simulink model "EM_3"  (R2016a)
settings: Solver=VariableStepAuto  StartTime=0.0  StopTime=0.12  RelTol=1e-3
settings Model: Creator=Максим  LastModifiedBy=Максим

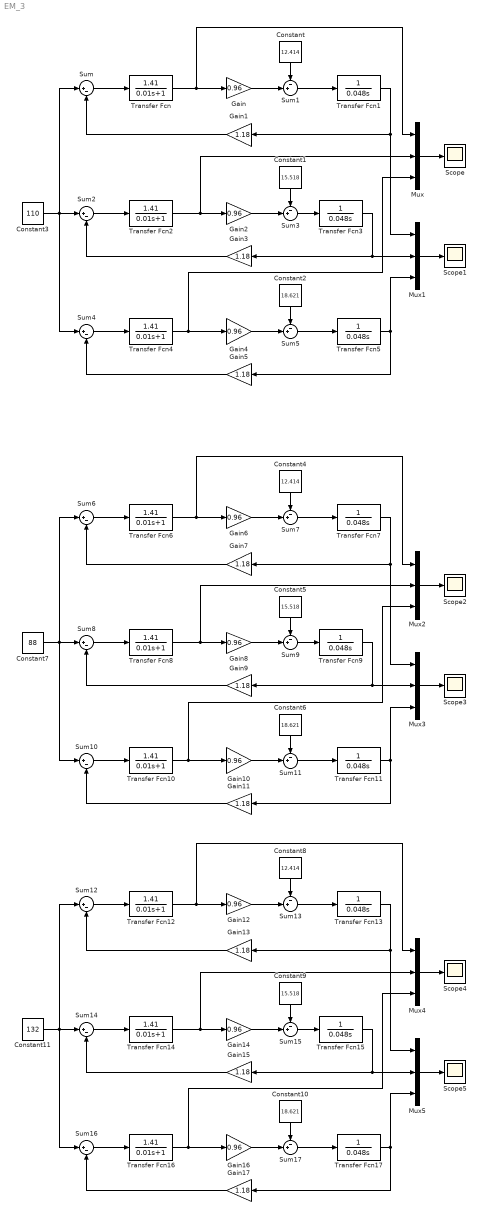
== system EM_3 ==
  Constant : Constant  Value=12.414
  Constant1 : Constant  Value=15.518
  Constant10 : Constant  Value=18.621
  Constant11 : Constant  Value=132
  Constant2 : Constant  Value=18.621
  Constant3 : Constant  Value=110
  Constant4 : Constant  Value=12.414
  Constant5 : Constant  Value=15.518
  Constant6 : Constant  Value=18.621
  Constant7 : Constant  Value=88
  Constant8 : Constant  Value=12.414
  Constant9 : Constant  Value=15.518
  Gain{,2,4,6,8,10,12,14,16} (9 alike) : Gain  Gain=0.96
  Gain{1,3,5,7,9,11,13,15,17} (9 alike) : Gain  Gain=1.18
  Mux{,1..5} (6 alike) : Mux  Inputs=3
  Scope{,1..5} (6 alike) : Scope
  Sum{,2,4,6,8,10,12,14,16} (9 alike) : Sum  Inputs=|+-
  Sum{1,3,5,7,9,11,13,15,17} (9 alike) : Sum  Inputs=-+|
  Transfer Fcn{,2,4,6,8,10,12,14,16} (9 alike) : TransferFcn  Numerator=[1.41]  Denominator=[0.01 1]
  Transfer Fcn{1,3,5,7,9,11,13,15,17} (9 alike) : TransferFcn  Denominator=[0.048 0]
  wires:
  Sum1/1 -> Transfer Fcn1/1
  Constant/1 -> Sum1/1
  Gain/1 -> Sum1/2
  Transfer Fcn/1 -> Mux/1, Gain/1
  Sum/1 -> Transfer Fcn/1
  Transfer Fcn1/1 -> Mux1/1, Gain1/1
  Gain1/1 -> Sum/2
  Sum3/1 -> Transfer Fcn3/1
  Constant1/1 -> Sum3/1
  Gain2/1 -> Sum3/2
  Transfer Fcn2/1 -> Mux/2, Gain2/1
  Sum2/1 -> Transfer Fcn2/1
  Transfer Fcn3/1 -> Mux1/2, Gain3/1
  Gain3/1 -> Sum2/2
  Sum5/1 -> Transfer Fcn5/1
  Constant2/1 -> Sum5/1
  Gain4/1 -> Sum5/2
  Transfer Fcn4/1 -> Mux/3, Gain4/1
  Sum4/1 -> Transfer Fcn4/1
  Transfer Fcn5/1 -> Gain5/1, Mux1/3
  Gain5/1 -> Sum4/2
  Constant3/1 -> Sum2/1, Sum/1, Sum4/1
  Mux/1 -> Scope/1
  Mux1/1 -> Scope1/1
  Sum7/1 -> Transfer Fcn7/1
  Constant4/1 -> Sum7/1
  Gain6/1 -> Sum7/2
  Transfer Fcn6/1 -> Mux2/1, Gain6/1
  Sum6/1 -> Transfer Fcn6/1
  Transfer Fcn7/1 -> Mux3/1, Gain7/1
  Gain7/1 -> Sum6/2
  Sum9/1 -> Transfer Fcn9/1
  Constant5/1 -> Sum9/1
  Gain8/1 -> Sum9/2
  Transfer Fcn8/1 -> Mux2/2, Gain8/1
  Sum8/1 -> Transfer Fcn8/1
  Transfer Fcn9/1 -> Mux3/2, Gain9/1
  Gain9/1 -> Sum8/2
  Sum11/1 -> Transfer Fcn11/1
  Constant6/1 -> Sum11/1
  Gain10/1 -> Sum11/2
  Transfer Fcn10/1 -> Mux2/3, Gain10/1
  Sum10/1 -> Transfer Fcn10/1
  Transfer Fcn11/1 -> Gain11/1, Mux3/3
  Gain11/1 -> Sum10/2
  Constant7/1 -> Sum8/1, Sum6/1, Sum10/1
  Mux2/1 -> Scope2/1
  Mux3/1 -> Scope3/1
  Sum13/1 -> Transfer Fcn13/1
  Constant8/1 -> Sum13/1
  Gain12/1 -> Sum13/2
  Transfer Fcn12/1 -> Mux4/1, Gain12/1
  Sum12/1 -> Transfer Fcn12/1
  Transfer Fcn13/1 -> Mux5/1, Gain13/1
  Gain13/1 -> Sum12/2
  Sum15/1 -> Transfer Fcn15/1
  Constant9/1 -> Sum15/1
  Gain14/1 -> Sum15/2
  Transfer Fcn14/1 -> Mux4/2, Gain14/1
  Sum14/1 -> Transfer Fcn14/1
  Transfer Fcn15/1 -> Mux5/2, Gain15/1
  Gain15/1 -> Sum14/2
  Sum17/1 -> Transfer Fcn17/1
  Constant10/1 -> Sum17/1
  Gain16/1 -> Sum17/2
  Transfer Fcn16/1 -> Mux4/3, Gain16/1
  Sum16/1 -> Transfer Fcn16/1
  Transfer Fcn17/1 -> Gain17/1, Mux5/3
  Gain17/1 -> Sum16/2
  Constant11/1 -> Sum14/1, Sum12/1, Sum16/1
  Mux4/1 -> Scope4/1
  Mux5/1 -> Scope5/1
